simulink model "chap11_4sim"  (Simulink 7.7)
settings: Solver=ode45  SolverMode=SingleTasking  StartTime=0.0  StopTime=30  FixedStep=0.001  RelTol=1e-3
settings Model: Creator=ljk  LastModifiedBy=ljk  ExtModeTrigMode=oneshot  ExtModeArmWhenConnect=off
settings DataIOCC: LimitDataPoints=off  SignalLoggingName=sigsOut
settings OptimizationCC: BooleanDataType=off
settings DebuggingCC: SaveWithParameterizedLinksMsg=none  SignalResolutionControl=TryResolveAllWithWarning  SolverPrmCheckMsg=none  MultiTaskDSMMsg=warning  MultiTaskCondExecSysMsg=none  StrictBusMsg=None
settings HardwareCC: TargetUnknown=on
settings RTWCC: IncludeERTFirstTime=on
settings CodeAppCC: CustomSymbolStrType=$N$R$M_T

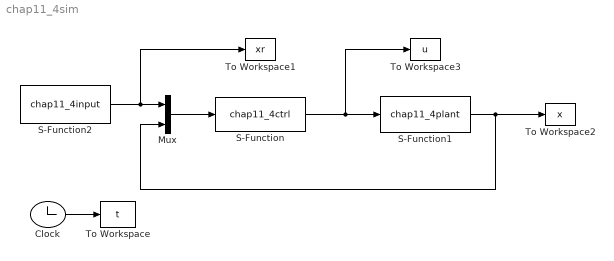
== system chap11_4sim ==
  Clock : Clock
  Mux : Mux  Inputs=2
  S-Function : S-Function  FunctionName=chap11_4ctrl  EnableBusSupport=off
  S-Function1 : S-Function  FunctionName=chap11_4plant  EnableBusSupport=off
  S-Function2 : S-Function  FunctionName=chap11_4input  EnableBusSupport=off
  To Workspace : ToWorkspace  VariableName=t  SampleTime=-1  SaveFormat=Array
  To Workspace1 : ToWorkspace  VariableName=xr  SampleTime=-1  SaveFormat=Array
  To Workspace2 : ToWorkspace  VariableName=x  SampleTime=-1  SaveFormat=Array
  To Workspace3 : ToWorkspace  VariableName=u  SampleTime=-1  SaveFormat=Array
  wires:
  Clock/1 -> To Workspace/1
  S-Function1/1 -> To Workspace2/1, Mux/2
  S-Function/1 -> S-Function1/1, To Workspace3/1
  S-Function2/1 -> Mux/1, To Workspace1/1
  Mux/1 -> S-Function/1
